simulink model "Modell_13_4_v2"  (R2018a)
settings: Solver=VariableStepAuto  StartTime=0.0  StopTime=20.0  RelTol=1e-3
InitFcn:
  | init_13_4
values from neighbouring files (symbols this model uses):
  a = 1    [init_13_1.m]    (also in init_13_1_v2.m; init_13_4.m)
  b = 1    [init.m]    (also in init_13_1.m; init_13_1_v2.m = 0.1111; init_13_4.m)
  c = 0.5    [init.m]    (also in init_13_1.m; init_13_1_v2.m = 0.8333; init_13_4.m = 1)
  kS = 1    [init_13_1_v2.m]    (also in init_13_4.m = 0.1)
  kT = 1    [init_13_1_v2.m]    (also in init_13_4.m)
  S01 = 30    [init_13_1_v2.m]    (also in init_13_4.m = 0.5)
  S02 = 35    [init_13_1_v2.m]    (also in init_13_4.m = 1)
  T01 = 29    [init_13_1_v2.m]    (also in init_13_4.m = 1)
  T02 = 12    [init_13_1_v2.m]    (also in init_13_4.m = 0.5)
  T1 = 10.8    [init_13_1_v2.m]
  T2 = 9.2    [init_13_1_v2.m]
settings Model: Creator=Uni  LastModifiedBy=ruedi

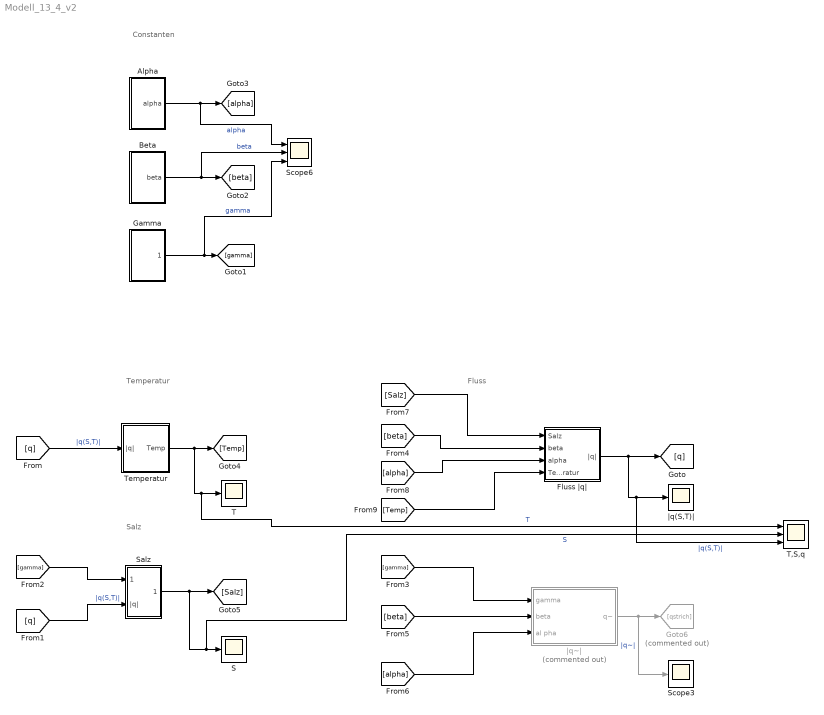
== system Modell_13_4_v2 ==
  note: Constanten
  note: Temperatur
  note: Salz
  note: Fluss
  Alpha : Subsystem
  Beta : Subsystem
  Fluss |q| : Subsystem
  Gamma : Subsystem
  Goto6 : Goto  Commented=on  GotoTag=qstrich
  S : Scope
  Salz : Subsystem
  Scope3 : Scope
  Scope6 : Scope  NumInputPorts=3
  T : Scope
  T,S,q : Scope  NumInputPorts=3
  Temperatur : Subsystem
  |q(S,T)| : Scope
  |q~| : Subsystem  Commented=on
  wires:
  Fluss |q|/1(|q|) -> T,S,q/3, |q(S,T)|/1, [q]  "|q(S,T)|"
  Gamma/1(gamma) -> Scope6/3, [gamma]  "gamma"
  |q~|/1(q~) -> Scope3/1, Goto6/1  "|q~|"
  [q] -> Salz/2(|q|)  "|q(S,T)|"
  [q] -> Temperatur/1(|q|)  "|q(S,T)|"
  [gamma] -> |q~|/1(gamma)
  [gamma] -> Salz/1(gamma)
  Beta/1(beta) -> Scope6/2, [beta]  "beta"
  [beta] -> Fluss |q|/2(beta)
  [beta] -> |q~|/2(beta)
  Alpha/1(alpha) -> Scope6/1, [alpha]  "alpha"
  [alpha] -> |q~|/3(al pha)
  Temperatur/1(Temp) -> T,S,q/1, T/1, [Temp]  "T"
  Salz/1("Salz ") -> T,S,q/2, S/1, [Salz]  "S"
  [Salz] -> Fluss |q|/1(Salz)
  [alpha] -> Fluss |q|/3(alpha)
  [Temp] -> Fluss |q|/4(Temperatur)

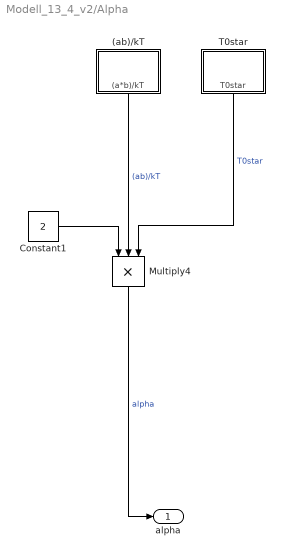
== system Modell_13_4_v2/Alpha ==
  (ab)/kT : Subsystem
  Constant1 : Constant  Value=2
  Multiply4 : Product  Inputs=3
  T0star : Subsystem
  alpha : Outport
  wires:
  (ab)/kT/1((a*b)/kT) -> Multiply4/2  "(ab)/kT"
  Multiply4/1 -> alpha/1  "alpha"
  T0star/1(T0star) -> Multiply4/3  "T0star"
  Constant1/1 -> Multiply4/1

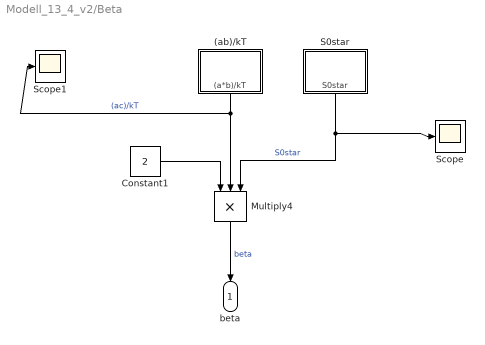
== system Modell_13_4_v2/Beta ==
  (ab)/kT : Subsystem
  Constant1 : Constant  Value=2
  Multiply4 : Product  Inputs=3
  S0star : Subsystem
  Scope : Scope
  Scope1 : Scope
  beta : Outport
  wires:
  Constant1/1 -> Multiply4/1
  S0star/1(S0star) -> Scope/1, Multiply4/3  "S0star"
  Multiply4/1 -> beta/1  "beta"
  (ab)/kT/1((a*b)/kT) -> Scope1/1, Multiply4/2  "(ac)/kT"

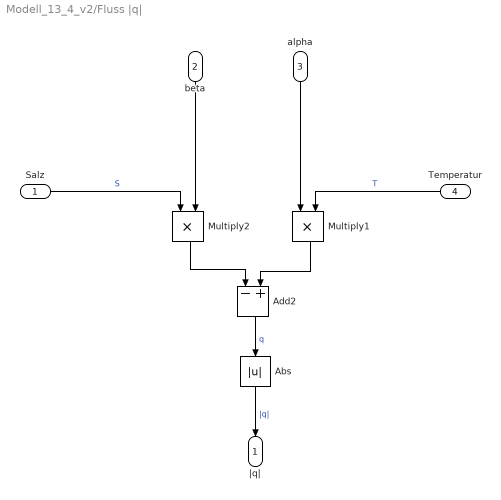
== system Modell_13_4_v2/Fluss |q| ==
  Salz : Inport
  beta : Inport  Port=2
  alpha : Inport  Port=3
  Temperatur : Inport  Port=4
  Abs : Abs
  Add2 : Sum  Inputs=-+
  Multiply1 : Product
  Multiply2 : Product
  |q| : Outport
  wires:
  Multiply2/1 -> Add2/1
  beta/1 -> Multiply2/2
  Temperatur/1 -> Multiply1/2  "T"
  Multiply1/1 -> Add2/2
  Abs/1 -> |q|/1  "|q|"
  Salz/1 -> Multiply2/1  "S"
  Add2/1 -> Abs/1  "q"
  alpha/1 -> Multiply1/1

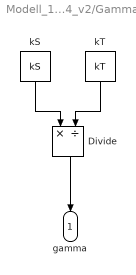
== system Modell_13_4_v2/Gamma ==
  Divide : Product  Inputs=*/
  kS : Constant  Value=kS
  kT : Constant  Value=kT
  gamma : Outport
  wires:
  kT/1 -> Divide/2
  kS/1 -> Divide/1
  Divide/1 -> gamma/1

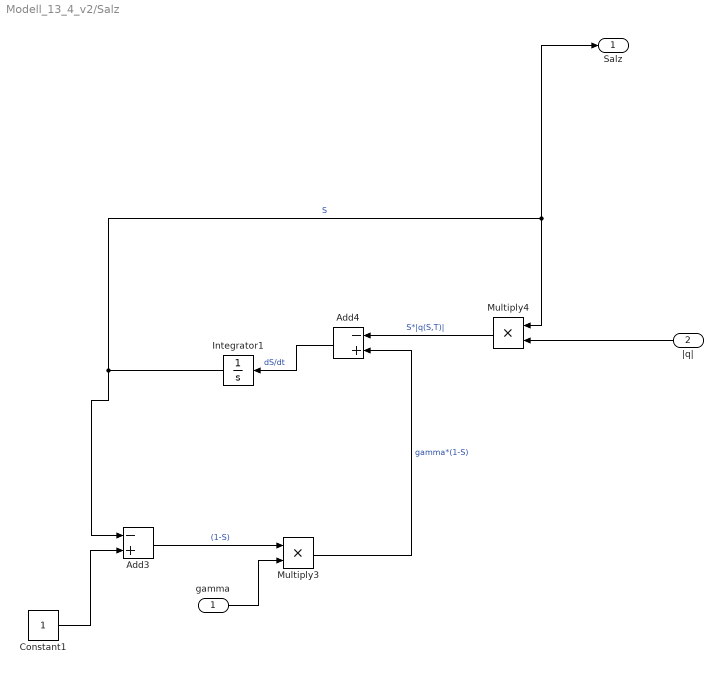
== system Modell_13_4_v2/Salz ==
  gamma : Inport
  |q| : Inport  Port=2
  Add3 : Sum  Inputs=-+
  Add4 : Sum  Inputs=-+
  Constant1 : Constant
  Integrator1 : Integrator  InitialCondition=1
  Multiply3 : Product
  Multiply4 : Product
  "Salz " : Outport
  wires:
  Multiply3/1 -> Add4/2  "gamma*(1-S)"
  Integrator1/1 -> Add3/1, "Salz "/1, Multiply4/1  "S"
  Add3/1 -> Multiply3/1  "(1-S)"
  Add4/1 -> Integrator1/1  "dS/dt"
  gamma/1 -> Multiply3/2
  Multiply4/1 -> Add4/1  "S*|q(S,T)|"
  Constant1/1 -> Add3/2
  |q|/1 -> Multiply4/2

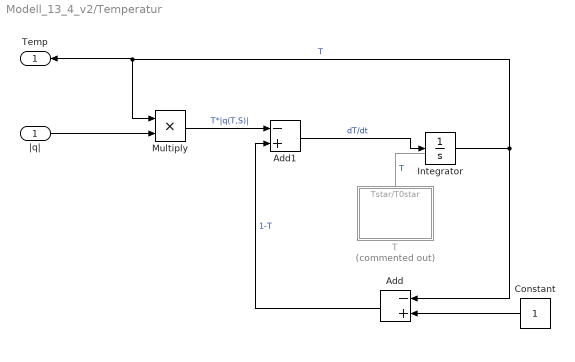
== system Modell_13_4_v2/Temperatur ==
  |q| : Inport
  Add : Sum  Inputs=-+
  Add1 : Sum  Inputs=-+
  Constant : Constant
  Integrator : Integrator  InitialCondition=1
  Multiply : Product
  T : Subsystem  Commented=on
  Temp : Outport
  wires:
  Integrator/1 -> Temp/1, Multiply/1, Add/1  "T"
  T/1(Tstar/T0star) -> ?  "T"
  Add/1 -> Add1/2  "1-T"
  |q|/1 -> Multiply/2
  Multiply/1 -> Add1/1  "T*|q(T,S)|"
  Constant/1 -> Add/2
  Add1/1 -> Integrator/1  "dT/dt"

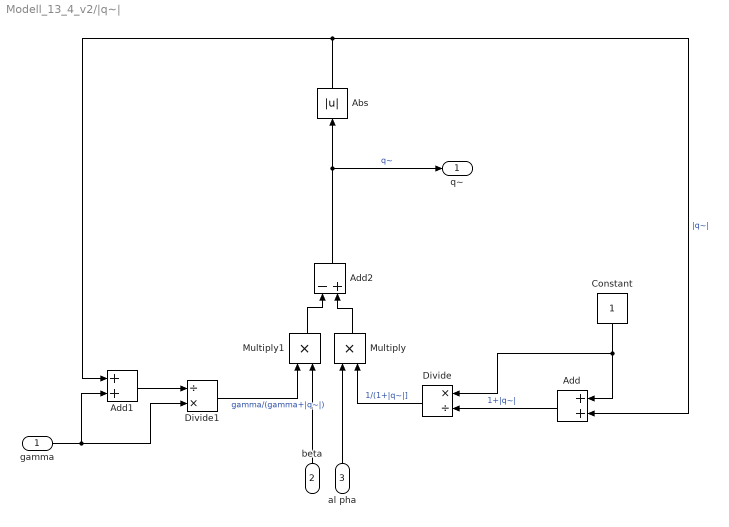
== system Modell_13_4_v2/|q~| ==
  gamma : Inport
  beta : Inport  Port=2
  al pha : Inport  Port=3
  Abs : Abs
  Add : Sum
  Add1 : Sum
  Add2 : Sum  Inputs=-+
  Constant : Constant
  Divide : Product  Inputs=*/
  Divide1 : Product  Inputs=/*
  Multiply : Product
  Multiply1 : Product
  q~ : Outport
  wires:
  gamma/1 -> Add1/2, Divide1/2
  Divide1/1 -> Multiply1/1  "gamma/(gamma+|q~|)"
  Abs/1 -> Add/2, Add1/1  "|q~|"
  Multiply/1 -> Add2/2
  Add1/1 -> Divide1/1
  Add2/1 -> Abs/1, q~/1  "q~"
  Add/1 -> Divide/2  "1+|q~|"
  Divide/1 -> Multiply/2  "1/(1+|q~|]"
  Multiply1/1 -> Add2/1
  beta/1 -> Multiply1/2
  al pha/1 -> Multiply/1
  Constant/1 -> Add/1, Divide/1

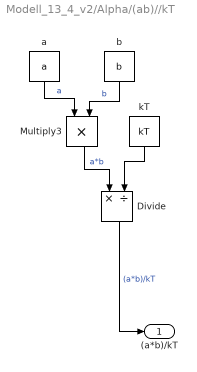
== system Modell_13_4_v2/Alpha/(ab)//kT ==
  Divide : Product  Inputs=*/
  Multiply3 : Product
  a : Constant  Value=a
  b : Constant  Value=b
  kT : Constant  Value=kT
  (a*b)/kT : Outport
  wires:
  b/1 -> Multiply3/2  "b"
  kT/1 -> Divide/2
  Multiply3/1 -> Divide/1  "a*b"
  Divide/1 -> (a*b)/kT/1  "(a*b)/kT"
  a/1 -> Multiply3/1  "a"

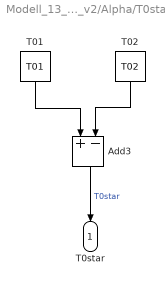
== system Modell_13_4_v2/Alpha/T0star ==
  Add3 : Sum  Inputs=+-
  T01 : Constant  Value=T01
  T02 : Constant  Value=T02
  T0star : Outport
  wires:
  T02/1 -> Add3/2
  T01/1 -> Add3/1
  Add3/1 -> T0star/1  "T0star"

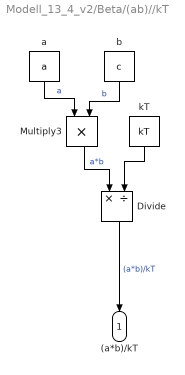
== system Modell_13_4_v2/Beta/(ab)//kT ==
  Divide : Product  Inputs=*/
  Multiply3 : Product
  a : Constant  Value=a
  b : Constant  Value=c
  kT : Constant  Value=kT
  (a*b)/kT : Outport
  wires:
  a/1 -> Multiply3/1  "a"
  Divide/1 -> (a*b)/kT/1  "(a*b)/kT"
  Multiply3/1 -> Divide/1  "a*b"
  kT/1 -> Divide/2
  b/1 -> Multiply3/2  "b"

== system Modell_13_4_v2/Beta/S0star ==
  Add3 : Sum  Inputs=+-
  S01 : Constant  Value=S01
  S02 : Constant  Value=S02
  S0star : Outport
  wires:
  Add3/1 -> S0star/1  "S0star"
  S01/1 -> Add3/1
  S02/1 -> Add3/2

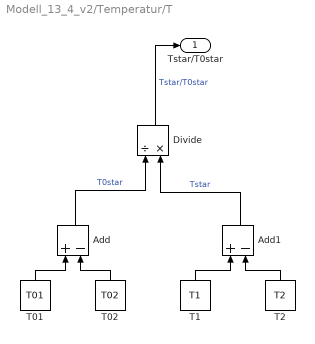
== system Modell_13_4_v2/Temperatur/T ==
  Add : Sum  Inputs=+-
  Add1 : Sum  Inputs=+-
  Divide : Product  Inputs=/*
  T01 : Constant  Value=T01
  T02 : Constant  Value=T02
  T1 : Constant  Value=T1
  T2 : Constant  Value=T2
  Tstar/T0star : Outport
  wires:
  Add/1 -> Divide/1  "T0star"
  T1/1 -> Add1/1
  Divide/1 -> Tstar/T0star/1  "Tstar/T0star"
  T02/1 -> Add/2
  Add1/1 -> Divide/2  "Tstar"
  T2/1 -> Add1/2
  T01/1 -> Add/1
